simulink model "sigma_delta_fxp"  (Simulink 7.7)
settings: Solver=FixedStepDiscrete  StartTime=0.0  StopTime=.02  FixedStep=1e-7  RelTol=1e-3
undefined symbols (not defined in the file or in its folder): dfilt, fdesignblkfcn, gcbh
libraries: simulink x1, dsparch4 x1
settings Model: Creator=embed  LastModifiedBy=embed
settings SolverCC: AutoInsertRateTranBlk=on
settings OptimizationCC: BlockReduction=off  ConditionallyExecuteInputs=off

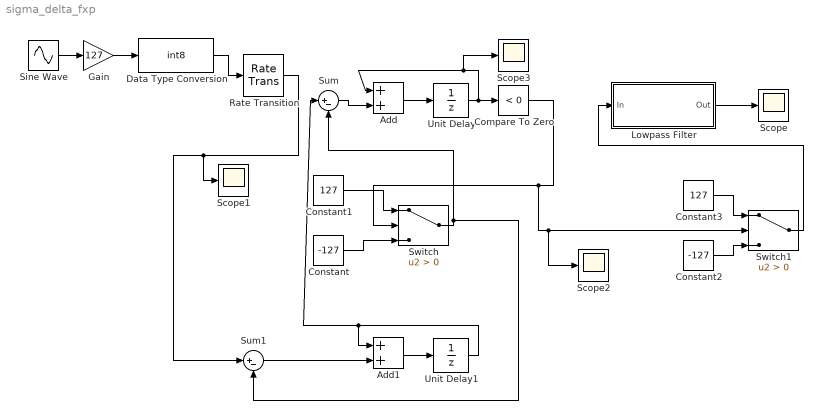
== system sigma_delta_fxp ==
  Add : Sum
  Add1 : Sum
  Compare To Zero : simulink/Logic and Bit Operations/Compare To Zero  SystemSampleTime=-1  relop=<  LogicOutDataTypeMode=boolean
  Constant : Constant  Value=-127  OutDataTypeStr=fixdt(1,25,7)
  Constant1 : Constant  Value=127  OutDataTypeStr=fixdt(1,25,7)
  Constant2 : Constant  Value=-127
  Constant3 : Constant  Value=127
  Data Type Conversion : DataTypeConversion  OutDataTypeStr=int8
  Gain : Gain  Gain=127
  Lowpass Filter : Subsystem  DialogController=fdesignblkfcn  DialogControllerArgs=DataTag1  InitFcn=fdesignblkfcn(gcbh, {'InitFcn'});
      settings: CopyFcn=fdesignblkfcn(gcbh, {'CopyFcn'});
      mask Type: Lowpass Filter
      mask Description: Design a lowpass filter
      mask Help: helpview(mapfilelocation('dsp'), 'dsplowpassfilter');
      mask Display: disp('Lowpass')
  Rate Transition : RateTransition  OutPortSampleTime=1e-7
  Scope{,1..3} (4 alike) : Scope
      Scope settings: MaxDataPoints=100000
      Scope1 settings: MaxDataPoints=100000
      Scope2 settings: SaveName=ScopeData2  MaxDataPoints=100000
      Scope3 settings: SaveName=ScopeData3  MaxDataPoints=100000
  Sine Wave : Sin  SineType=Sample based  Samples=195  SampleTime=512/10e6
  Sum : Sum  Inputs=|+-  SampleTime=1e-7
  Sum1 : Sum  Inputs=|+-  OutDataTypeStr=fixdt(1,25,7)  SampleTime=1e-7
  Switch : Switch  Criteria=u2 > Threshold
  Switch1 : Switch  Criteria=u2 > Threshold  OutDataTypeStr=Inherit: Inherit via back propagation
  Unit Delay : UnitDelay  SampleTime=-1
  Unit Delay1 : UnitDelay  SampleTime=-1
  wires:
  Compare To Zero/1 -> Switch/2, Switch1/2, Scope2/1
  Switch/1 -> Sum/2, Sum1/2
  Constant1/1 -> Switch/1
  Constant/1 -> Switch/3
  Unit Delay/1 -> Compare To Zero/1, Add/1, Scope3/1
  Sum/1 -> Add/2
  Add/1 -> Unit Delay/1
  Lowpass Filter/1(Out) -> Scope/1
  Sine Wave/1 -> Gain/1
  Gain/1 -> Data Type Conversion/1
  Data Type Conversion/1 -> Rate Transition/1
  Constant3/1 -> Switch1/1
  Constant2/1 -> Switch1/3
  Switch1/1 -> Lowpass Filter/1(In)
  Unit Delay1/1 -> Add1/1, Sum/1
  Add1/1 -> Unit Delay1/1
  Rate Transition/1 -> Scope1/1, Sum1/1
  Sum1/1 -> Add1/2

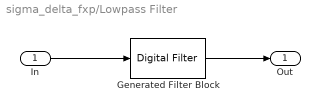
== system sigma_delta_fxp/Lowpass Filter ==
  In : Inport
  Generated Filter Block : dsparch4/Digital Filter  Tag=BlockMethodSubSystem  TypePopup=FIR (all zeros)  IIRFiltStruct=Direct form II transposed  AllPoleFiltStruct=Direct form  FIRFiltStruct=Direct form  CoeffSource=Specify via dialog  NumCoeffs=[-0.00122653615946103 -0.000261599293671628 -0.000287838427665307 -0.000314631376729338 -0.000341745179896497 -0.000368970388904827 -0.000396091245541113 -0.000422918477294773 -0.000449183855943477 -0.000474639710638397 -0.000499110369506131 -0.000522284360425836 -0.000543881771761834 -0.000563688747445864 -0.000581253427601942 -0.000596241836396328 -0.000608251671564388 -0.000616875059714026 -0.000621857986331903 -0.000622744601161802 -0.000619372039332745 -0.000611416659994283 -0.000598403231281537 -0.00057987030389329 -0.000555176987171597 -0.000523721250674614 -0.000485328335365384 -0.000440248160236351 -0.000388574746872102 -0.000328850992818485 -0.00025812652261886 -0.000182398529454224 -9.57474756453213e-005 -3.7927927853563e-007 0.000104570993323406 0.000219310147224563 0.000344075637675361 0.000479149714201888 0.000624729242326618 0.000781007085812387 0.000948193761101985 0.00112632708415366 0.00131547043723616 0.0015157410569676 0.00172708366546137 0.00194953455469662 0.00218307734880749 0.00242759272602341 0.00268309064417582 0.00294911942948531 0.0032256032473754 0.00351223488169483 0.00380870798584049 0.00411490666143474 0.00443045009418711 0.00475468190697462 0.00508703143350159 0.00542724842853343 0.00577515642652566 0.00612978280522486 0.00648986529659215 0.00685638067408811 0.00722720989679994 0.00760243415105599 0.007981040730859 0.00836231620806653 0.00874550420104979 0.00912978052783701 0.00951437255763479 0.00989844459488267 0.0102810829154739 0.0106614829836345 0.0110387602889876 0.0114119598610684 0.0117802571730694 0.0121427700204889 0.0124986245925902 0.0128470344762918 0.0131868634296189 0.0135175972728676 0.0138380749853982 0.0141476455373706 0.01444565905604 0.0147311217371358 0.015003209472129 0.015261369831249 0.0155050544351962 0.0157334780630414 0.015945769048561 0.0161415969444687 0.0163207280215537 0.016482005406953 0.0166256219589734 0.0167507794479614 0.0168572985397198 0.0169448638791241 0.0170132126275138 0.0170621882927403 0.0170916061431394 0.0171013978330292 0.0170916061431394 0.0170621882927403 0.0170132126275138 0.0169448638791241 0.0168572985397198 0.0167507794479614 0.0166256219589734 0.016482005406953 0.0163207280215537 0.0161415969444687 0.015945769048561 0.0157334780630414 0.0155050544351962 0.015261369831249 0.015003209472129 0.0147311217371358 0.01444565905604 0.0141476455373706 0.0138380749853982 0.0135175972728676 0.0131868634296189 0.0128470344762918 0.0124986245925902 0.0121427700204889 0.0117802571730694 0.0114119598610684 0.0110387602889876 0.0106614829836345 0.0102810829154739 0.00989844459488267 0.00951437255763479 0.00912978052783701 0.00874550420104979 0.00836231620806653 0.007981040730859 0.00760243415105599 0.00722720989679994 0.00685638067408811 0.00648986529659215 0.00612978280522486 0.00577515642652566 0.00542724842853343 0.00508703143350159 0.00475468190697462 0.00443045009418711 0.00411490666143474 0.00380870798584049 0.00351223488169483 0.0032256032473754 0.00294911942948531 0.00268309064417582 0.00242759272602341 0.00218307734880749 0.00194953455469662 0.00172708366546137 0.0015157410569676 0.00131547043723616 0.00112632708415366 0.000948193761101985 0.000781007085812387 0.000624729242326618 0.000479149714201888 0.000344075637675361 0.000219310147224563 0.000104570993323406 -3.7927927853563e-007 -9.57474756453213e-005 -0.000182398529454224 -0.00025812652261886 -0.000328850992818485 -0.000388574746872102 -0.000440248160236351 -0.000485328335365384 -0.000523721250674614 -0.000555176987171597 -0.00057987030389329 -0.000598403231281537 -0.000611416659994283 -0.000619372039332745 -0.000622744601161802 -0.000621857986331903 -0.000616875059714026 -0.000608251671564388 -0.000596241836396328 -0.000581253427601942 -0.000563688747445864 -0.000543881771761834 -0.000522284360425836 -0.000499110369506131 -0.000474639710638397 -0.000449183855943477 -0.000422918477294773 -0.000396091245541113 -0.000368970388904827 -0.000341745179896497 -0.000314631376729338 -0.000287838427665307 -0.000261599293671628 -0.00122653615946103]  DenCoeffs=[1 0.1]  BiQuadCoeffs=[1 0.3 0.4 1 0.1 0.2]  LatticeCoeffs=[0.2 0.4]  denIgnore=on  FiltPerSampPopup=One filter per frame  IC=0  ICnum=0  ICden=0  roundingMode=Floor  overflowMode=off  ScaleValues=1  scaleValueFracLength=14  stageInFracLength=15  stageOutFracLength=15  FilterSource=Specify via dialog  dfiltObjectName=dfilt.dffir([1 2 1])  InputProcessing=Columns as channels (frame based)
  Out : Outport
  wires:
  In/1 -> Generated Filter Block/1
  Generated Filter Block/1 -> Out/1
